simulink model "linearizedUnicycleRobotDynamics"  (R2016a)
settings: Solver=VariableStepAuto  StartTime=0.0  StopTime=10.0  RelTol=1e-3
libraries: simulink x1
settings Model: Creator=jagni  LastModifiedBy=jagni

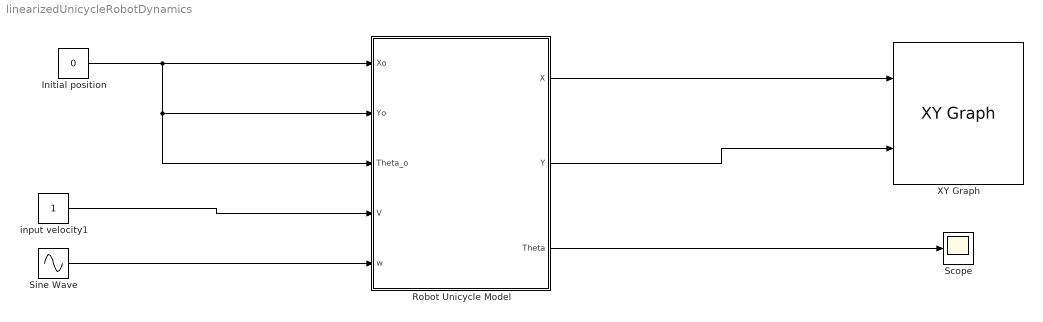
== system linearizedUnicycleRobotDynamics ==
  "Initial position " : Constant  Value=0
  "Robot Unicycle Model " : Subsystem
  Scope : Scope
  Sine Wave : Sin  Frequency=.01  SampleTime=0
  XY Graph : simulink/Sinks/XY Graph  xmin=-10  xmax=10  ymin=-10  ymax=10  st=-1
  input velocity1 : Constant
  wires:
  "Initial position "/1 -> "Robot Unicycle Model "/3(Theta_o), "Robot Unicycle Model "/2(Yo), "Robot Unicycle Model "/1(Xo)
  input velocity1/1 -> "Robot Unicycle Model "/4(V)
  Sine Wave/1 -> "Robot Unicycle Model "/5(w)
  "Robot Unicycle Model "/1(X) -> XY Graph/1
  "Robot Unicycle Model "/2(Y) -> XY Graph/2
  "Robot Unicycle Model "/3("Theta ") -> Scope/1

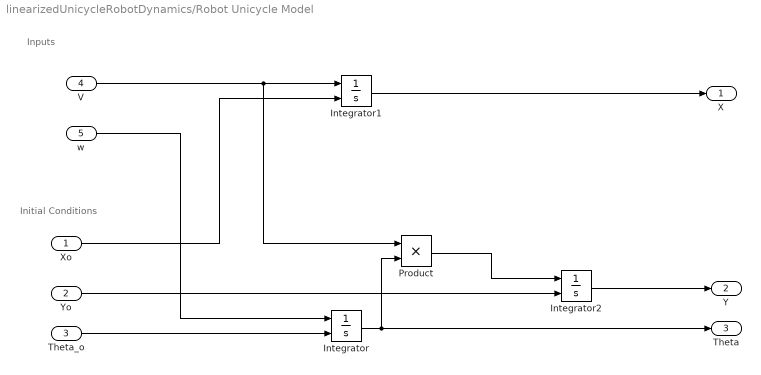
== system linearizedUnicycleRobotDynamics/Robot Unicycle Model  ==
  note: Inputs
  note: Initial Conditions
  Xo : Inport
  Yo : Inport  Port=2
  Theta_o : Inport  Port=3
  V : Inport  Port=4
  w : Inport  Port=5
  Integrator : Integrator  InitialConditionSource=external
  Integrator1 : Integrator  InitialConditionSource=external
  Integrator2 : Integrator  InitialConditionSource=external
  Product : Product
  X : Outport
  Y : Outport  Port=2
  "Theta " : Outport  Port=3
  wires:
  Theta_o/1 -> Integrator/2
  w/1 -> Integrator/1
  Xo/1 -> Integrator1/2
  Integrator1/1 -> X/1
  V/1 -> Product/1, Integrator1/1
  Integrator/1 -> Product/2, "Theta "/1
  Yo/1 -> Integrator2/2
  Product/1 -> Integrator2/1
  Integrator2/1 -> Y/1
